simulink model "Part1"  (R2020a)
settings: Solver=VariableStepAuto  StartTime=0.0  StopTime=200  RelTol=1e-3
values from neighbouring files (symbols this model uses):
  b = 50    [Script1.m]
  Force = 1250    [Script1.m]
  m = 1000    [Script1.m]
libraries: cstblocks x1
settings Model: Creator=maxen  LastModifiedBy=maxen

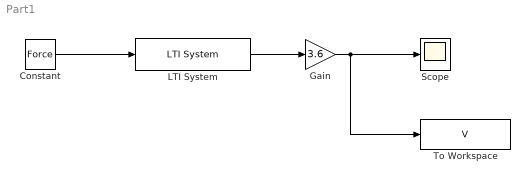
== system Part1 ==
  Constant : Constant  Value=Force
  Gain : Gain  Gain=3.6
  LTI System : cstblocks/LTI System  sys=tf(1,[m b])  IC=[]
  Scope : Scope
  To Workspace : ToWorkspace  VariableName=V  SampleTime=-1
  wires:
  Constant/1 -> LTI System/1
  LTI System/1 -> Gain/1
  Gain/1 -> To Workspace/1, Scope/1
